simulink model "mavsim_chap4"  (R2017a)
settings: Solver=ode45  StartTime=0.0  StopTime=999  RelTol=1e-3  EnableMultiTasking=on
InitFcn:
  | param_chap4
undefined symbols (not defined in the file or in its folder): airdata, drawAircraft, plotmavstatevariables, traj_line
libraries: simulink x4
settings Model: Creator=beard  LastModifiedBy=STAN
settings DataIOCC: LimitDataPoints=on  SaveFormat=Array  SignalLoggingSaveFormat=ModelDataLogs
settings OptimizationCC: ExpressionDepthLimit=2147483647  InitFltsAndDblsToZero=on  LifeSpan=inf
settings DebuggingCC: UnderspecifiedInitializationDetection=Classic  MergeDetectMultiDrivingBlocksExec=none  SolverPrmCheckMsg=warning  FcnCallInpInsideContextMsg=warning  StateNameClashWarn=warning  SFUnexpectedBacktrackingDiag=warning  SFNoUnconditionalDefaultTransitionDiag=warning  SFExecutionAtInitializationDiag=none
settings HardwareCC: ProdBitPerPointer=32  ProdBitPerSizeT=32  ProdBitPerPtrDiffT=32  ProdLargestAtomicFloat=None  ProdIntDivRoundTo=Undefined  ProdEndianess=Unspecified  ProdWordSize=32  ProdHWDeviceType=32-bit Generic
settings ModelReferenceCC: PropagateSignalLabelsOutOfModel=off
settings GRTTargetCC: TargetLangStandard=C89/C90 (ANSI)  GeneratePreprocessorConditionals=Disable all  CombineOutputUpdateFcns=off  GRTInterface=on
settings ConfigComp: CovMetricSettings=dw  CovHtmlReporting=on  CovSaveCumulativeToWorkspaceVar=on  CovSaveSingleToWorkspaceVar=on  CovExternalEMLEnable=off  CovSFcnEnable=off

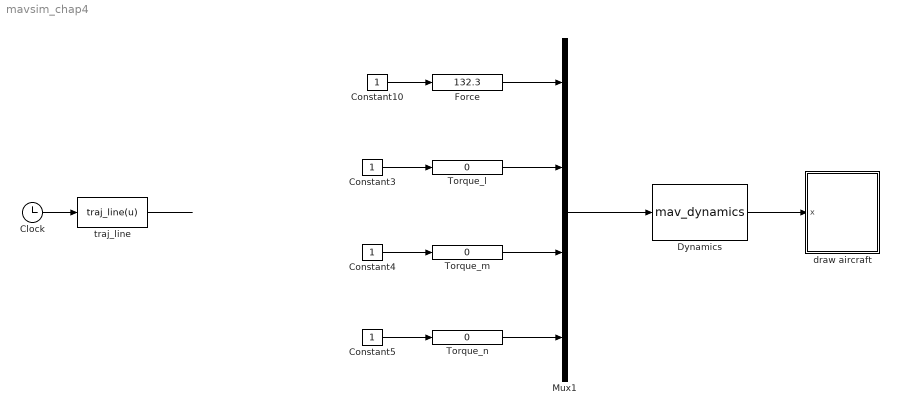
== system mavsim_chap4 ==
  Clock : Clock
  Constant{3..5,10} (4 alike) : Constant
  Dynamics : S-Function  FunctionName=mav_dynamics  Parameters=P  SFunctionDeploymentMode=off  EnableBusSupport=off
  Force : simulink/Math Operations/Slider Gain  gain=132.3  low=-100  high=150
  Mux1 : Mux
  Torque_l : simulink/Math Operations/Slider Gain  gain=0  low=-1  high=1
  Torque_m : simulink/Math Operations/Slider Gain  gain=0  low=-100  high=100
  "Torque_n " : simulink/Math Operations/Slider Gain  gain=0  low=-100  high=100
  draw aircraft : Subsystem
      mask Display: image(imread('tv.jpg'))
  traj_line : MATLABFcn  MATLABFcn=traj_line(u)  OutputDimensions=11
  wires:
  Constant5/1 -> "Torque_n "/1
  Constant10/1 -> Force/1
  Dynamics/1 -> draw aircraft/1(x)
  Force/1 -> Mux1/1
  "Torque_n "/1 -> Mux1/4
  Constant4/1 -> Torque_m/1
  Torque_m/1 -> Mux1/3
  Constant3/1 -> Torque_l/1
  Torque_l/1 -> Mux1/2
  Mux1/1 -> Dynamics/1
  Clock/1 -> traj_line/1
  traj_line/1 -> ?

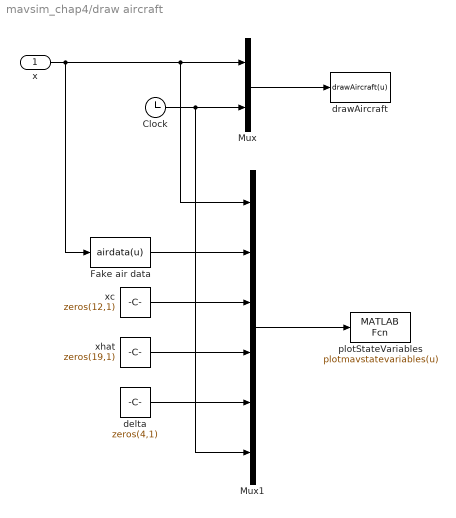
== system mavsim_chap4/draw aircraft ==
  x : Inport
  Clock : Clock
  Fake air data : MATLABFcn  MATLABFcn=airdata(u)  OutputDimensions=6  SampleTime=0.1
  Mux : Mux  Inputs=2
  Mux1 : Mux  Inputs=6
  delta : Constant  Value=zeros(4,1)
  drawAircraft : MATLABFcn  MATLABFcn=drawAircraft(u)  OutputDimensions=0  SampleTime=0.1
  plotStateVariables : MATLABFcn  MATLABFcn=plotmavstatevariables(u)  OutputDimensions=0  SampleTime=0.1
  xc : Constant  Value=zeros(12,1)
  xhat : Constant  Value=zeros(19,1)
  wires:
  Mux/1 -> drawAircraft/1
  x/1 -> Mux/1, Mux1/1, Fake air data/1
  Clock/1 -> Mux/2, Mux1/6
  Mux1/1 -> plotStateVariables/1
  xhat/1 -> Mux1/4
  xc/1 -> Mux1/3
  delta/1 -> Mux1/5
  Fake air data/1 -> Mux1/2
